simulink model "ParkTran"  (R2022b)
settings: Solver=FixedStepDiscrete  StartTime=0.0  StopTime=10.0  FixedStep=0.000001  RelTol=1e-3
settings Model: Creator=yll  LastModifiedBy=yll

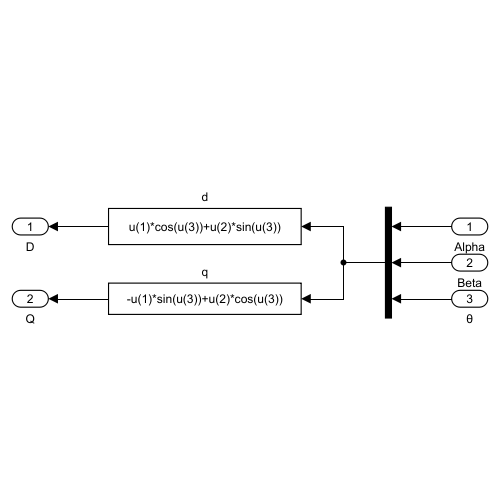
[thumbnail: Simulink's stored preview of the top-level diagram]
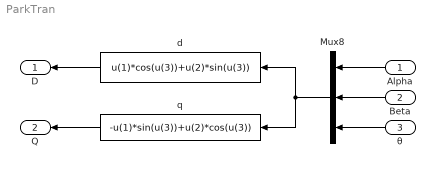
== system ParkTran ==
  Alpha : Inport
  Beta : Inport  Port=2
  θ : Inport  Port=3
  " d" : Fcn  Expr=u(1)*cos(u(3))+u(2)*sin(u(3))
  " q" : Fcn  Expr=-u(1)*sin(u(3))+u(2)*cos(u(3))
  Mux8 : Mux  Inputs=3
  D : Outport
  Q : Outport  Port=2
  wires:
  Beta/1 -> Mux8/2
  Alpha/1 -> Mux8/1
  θ/1 -> Mux8/3
  Mux8/1 -> " q"/1, " d"/1
  " d"/1 -> D/1
  " q"/1 -> Q/1
